simulink subsystem "ConvertToTheta"  (R2024a)
settings: Solver=VariableStepAuto  StartTime=0.0  StopTime=10.0  RelTol=1e-3
undefined symbols (not defined in the file or in its folder): dx
libraries: simulink x1
settings Model: Creator=44779  LastModifiedBy=44779

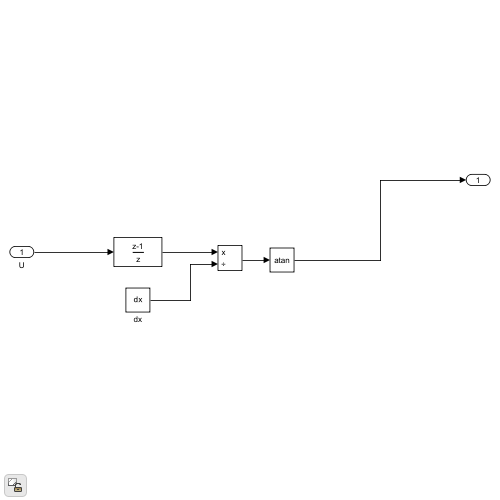
[thumbnail: Simulink's stored preview of the top-level diagram]
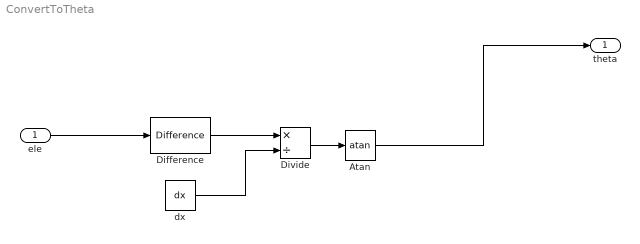
== system ConvertToTheta ==
  ele : Inport
  Atan : Trigonometry  Operator=atan
  Difference : simulink/Discrete/Difference  ICPrevInput=0.0  OutMin=[]  OutMax=[]  OutDataType=fixdt(1, 16)  OutScaling=2^-10  DoSatur=off
  Divide : Product  Inputs=*/
  dx : Constant  Value=dx
  theta : Outport
  wires:
  Difference/1 -> Divide/1
  Atan/1 -> theta/1
  dx/1 -> Divide/2
  Divide/1 -> Atan/1
  ele/1 -> Difference/1
